simulink model "Test_Aekf"  (R2025b)
settings: Solver=VariableStepAuto  StartTime=0.0  StopTime=StopTime  RelTol=1e-3
undefined symbols (not defined in the file or in its folder): batt
settings Model: Creator=faxio  LastModifiedBy=faxio

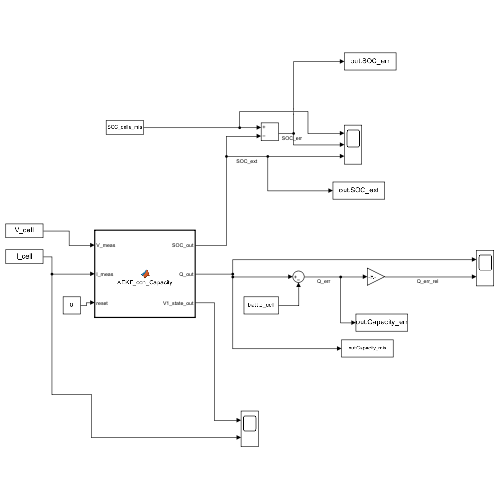
[thumbnail: Simulink's stored preview of the top-level diagram]
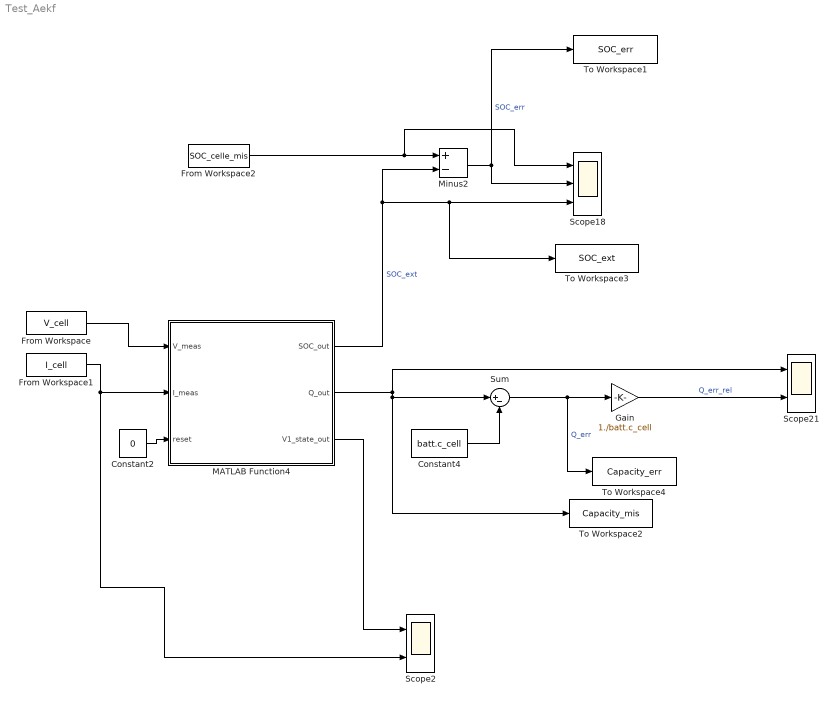
== system Test_Aekf ==
  Constant2 : Constant  Value=0
  Constant4 : Constant  Value=batt.c_cell
  From Workspace : FromWorkspace  VariableName=V_cell
  From Workspace1 : FromWorkspace  VariableName=I_cell
  From Workspace2 : FromWorkspace  VariableName=SOC_celle_mis
  Gain : Gain  Gain=1./batt.c_cell
  MATLAB Function4 : MATLAB Function  TreatAsAtomicUnit=on
  Minus2 : Sum  Inputs=+-
  Scope18 : Scope  NumInputPorts=3
      settings: ActiveDisplayYMinimum=-0.012590051184695097  ActiveDisplayYMaximum=1.1125100056871884  DataLoggingVariableName=ScopeData18
  Scope2 : Scope  NumInputPorts=2
      settings: ActiveDisplayYMinimum=-0.38132934403952395  ActiveDisplayYMaximum=0.3863878602749713
  Scope21 : Scope  NumInputPorts=2
      settings: ActiveDisplayYMinimum=55.008001380546148  ActiveDisplayYMaximum=58.3341308269945  DataLoggingVariableName=ScopeData21
  Sum : Sum  Inputs=|+-
  To Workspace1 : ToWorkspace  VariableName=SOC_err  SaveFormat=Timeseries  SampleTime=-1
  To Workspace2 : ToWorkspace  VariableName=Capacity_mis  SaveFormat=Timeseries  SampleTime=-1
  To Workspace3 : ToWorkspace  VariableName=SOC_ext  SaveFormat=Timeseries  SampleTime=-1
  To Workspace4 : ToWorkspace  VariableName=Capacity_err  SaveFormat=Timeseries  SampleTime=-1
  wires:
  Sum/1 -> To Workspace4/1, Gain/1  "Q_err"
  MATLAB Function4/2(Q_out) -> Scope21/1, To Workspace2/1, Sum/1
  Constant4/1 -> Sum/2
  Constant2/1 -> MATLAB Function4/3(reset)
  MATLAB Function4/1(SOC_out) -> Minus2/2, Scope18/3, To Workspace3/1  "SOC_ext"
  Minus2/1 -> To Workspace1/1, Scope18/2  "SOC_err"
  From Workspace/1 -> MATLAB Function4/1(V_meas)
  From Workspace1/1 -> Scope2/2, MATLAB Function4/2(I_meas)
  From Workspace2/1 -> Scope18/1, Minus2/1
  Gain/1 -> Scope21/2  "Q_err_rel"
  MATLAB Function4/3(V1_state_out) -> Scope2/1

== matlab function Test_Aekf/MATLAB Function4 ==
  settings: updateMethod=DISCRETE  sampleTime=0.5
  data: SOC_out output; Q_out output; V_meas input; I_meas input; reset input; batt_param parameter; V1_state_out output
function [SOC_out, Q_out,V1_state_out]   = AEKF_con_Capacity(V_meas, I_meas, reset,batt_param)  %#codegen

% Ingressi:
%   V_meas - Vettore tensioni misurate [n_cells x 1]
%   I_meas - Vettore correnti misurate [n_cells x 1]  
%   reset  - Segnale di reset (booleano)
%
% Uscita:
%   SOC_out - SOC stimato [n_cells x 1]
%   Q_out   - Capacità stimata [n_cells x 1]


    M=50; %finestra di misura per AEKF
    % Numero di celle 
    n_cells = 4;

    % Parametri batteria
    Ts = 0.5;           % Tempo campionamento [s]
    Q_cell = batt_param.c_cell;        % Capacità nominale [Ah]
    R0_matrix = batt_param.r0;         % Resistenza ohmica [Ohm]
    R1_matrix = batt_param.r1;         % Resistenza RC [Ohm]
    C1_matrix = batt_param.c1;          % Capacità RC [F]
    
    SOC_grid =batt_param.soc(:);
    OCV_tab  =batt_param.ocv(:);
    dOCV_tab =batt_param.docv(:);

    % % Rumore EKF
    % Q_cov = diag([1e-5, 1e-3, 1e-8]);
    % R_var = 0.00001;
    
    persistent SOC_state V1_state Q_state P_state H_k_vector Q_cov R_var initialized 
    persistent I_prev %variabile messa per salvare la corrente precedente e verificare se ci sono picchi di corrente

        if isempty(I_prev)
        I_prev = zeros(n_cells, 1);
        end

    if isempty(initialized) || reset
        SOC_state = 0.5 * ones(n_cells,1);
        V1_state  = zeros(n_cells,1);
        Q_state   = Q_cell(:); % inizializza con capacità nominale
        P_state   = zeros(3,3,n_cells);
    
        %inizializziamo i parametri, uno per ogni cella
        H_k_vector = NaN(n_cells, M); 
        Q_cov = zeros(3, 3, n_cells); 
        R_var = zeros(n_cells, 1);   
    
        for k = 1:n_cells
            P_state(:,:,k) = diag([0.05, 0.01, 1e-3]);

            Q_cov(:,:,k) = diag([1e-5, 1e-3, 1e-10]); % rumore piccolo inizialmente su Q (variazione lenta)
            R_var(k) = 0.00001;
        end
        initialized = true;
    end

    %% PRE-ALLOCAZIONE

    SOC_out = zeros(n_cells,1);
    Q_out   = zeros(n_cells,1);

    V1_state_out= zeros(n_cells,1);


    %% EKF PER OGNI CELLA

    for k = 1:n_cells

        % Stato corrente
        x = [SOC_state(k); V1_state(k); Q_state(k)];
        P = P_state(:,:,k);

        Q_cov_k = Q_cov(:,:,k);  
        R_var_k = R_var(k);

        I_k = I_meas(k);
        V_k = V_meas(k);

        %% PREDIZIONE 
        % Coulomb counting
        Q_k = max(1e-6, x(3)); % fa evitare divisione per zero
        SOC_pred = x(1) - (Ts * I_k) / (Q_k * 3600);
        SOC_pred = max(0.1, min(1, SOC_pred)); %limito il soc tra 0.1 e 1
    
        % ESTRAGGO LA RIGA k DALLA MATRICE E FACCIO L'INTERPOLAZIONE
        R0_row = R0_matrix(k, :);  % Riga k, vettore [1 x 21]
        R1_row = R1_matrix(k, :);  % Riga k, vettore [1 x 21]
        C1_row = C1_matrix(k, :);  % Riga k, vettore [1 x 21]
        
        % Converte a colonna per interp1
        R0_col = R0_row(:);  % [21 x 1]
        R1_col = R1_row(:);  % [21 x 1]
        C1_col = C1_row(:);  % [21 x 1]

        % Interpolazione
        R0 = interp1(SOC_grid, R0_col, SOC_pred, 'linear', 'extrap');
        R1 = interp1(SOC_grid, R1_col, SOC_pred, 'linear', 'extrap');
        C1 = interp1(SOC_grid, C1_col, SOC_pred, 'linear', 'extrap');
    
        R0=R0/Q_k*Q_cell(k);
        R1=R1/Q_k*Q_cell(k);
        C1=C1*Q_k/Q_cell(k);

        tau1  = R1 * C1;
        alpha = exp(-Ts / tau1);

        % Dinamica RC
        V1_pred = alpha * x(2) + R1 * (1 - alpha) * I_k;

        % Q pred
        Q_pred = x(3);

        x_pred = [SOC_pred; V1_pred; Q_pred];

        % Jacobiano stato
        dSOCdQ = (Ts * I_k) / (Q_k^2 * 3600);
        A =[1, 0, dSOCdQ;
            0, alpha, 0;
            0, 0, 1];
        
        %% ///////////////////////////////////
        % inserisco una condizione che verifica che la derivata della
        % corrente non sia molto alta, nel caso in cui lo fosse Q_cov va
        % aumentato. Ho aggiunto come persistent Iprev
        

        % Rileviamo la variazione di corrente
        dI = abs(I_k - I_prev(k));

        if dI > 0.3 * Q_cell(k)  % Impulso rilevato
            Q_cov_k_temp = Q_cov_k;
            Q_cov_k_temp(1,1) = Q_cov_k(1,1) * 100;
            Q_cov_k_temp(2,2) = Q_cov_k(2,2) * 50;  
            % Q(3,3) rimane uguale (variazione di capacità lenta)
        else
            Q_cov_k_temp = Q_cov_k;  %// Usa valore normale
        end

        P_pred = A * P * A' + Q_cov_k_temp;

        I_prev(k) = I_k;

        %////////////////////////////////////////
        %% AGGIORNAMENTO
        OCV  = interp1(SOC_grid, OCV_tab, SOC_pred,"linear","extrap");
        dOCV = interp1(SOC_grid, dOCV_tab, SOC_pred,"linear","extrap");
        
        V_pred = OCV - x_pred(2) - R0 * I_k;
        y_tilde = V_k - V_pred;
    
        %liomitiamo per swicurezza anche y_tilde soprattutto ad alte correnti
        C_rate = abs(I_k) / Q_cell(k);
        if C_rate > 1.5
            y_tilde = max(-0.1, min(0.1, y_tilde));
        else
            y_tilde = max(-0.8, min(0.8, y_tilde));
        end

        C_mat = [dOCV, -1, 0];

        S = C_mat * P_pred * C_mat' + R_var_k;
        K = (P_pred * C_mat') / S;
        
        % Possiamo pensare di inserire una protezione sulla stima della
        % capacità per far in modo che venga più precisa mettendo dei
        % limitti su quando stimarla.

        % Condizioni per NON aggiornare Q:
        disable_Q_update = false;

        % 1. Corrente troppo bassa (< 0.1C)
        if abs(I_k) < 0.1 * Q_cell(k)
            disable_Q_update = true;
        end

        % 2. Picchi di corrente
        if dI > 0.3 * Q_cell(k)
            disable_Q_update = true;
        end

        % 3. SOC estremi (modello impreciso)
        if SOC_pred < 0.15 || SOC_pred > 0.85
            disable_Q_update = true;
        end

        % 4. Innovazione troppo grande (modello sbagliato)
        if abs(y_tilde) > 0.1
            disable_Q_update = true;
        end

        % Azzera K(3) se le condizioni non sono buone
        if disable_Q_update
            K(3) = 0; 
        end
        %%

        % Aggiornamento stato
        x_upd = x_pred + K * y_tilde;
        x_upd(1) = max(0.05, min(1, x_upd(1)));
        x_upd(3) = max(1e-6, x_upd(3)); % capacità sempre positiva

        % Aggiornamento covarianza
        I3 = eye(3);
        P_upd = (I3 - K * C_mat) * P_pred;

        % Forziamo la simmetria
        P_upd = (P_upd + P_upd') / 2;

        H_k_vector(k,:)=circshift(H_k_vector(k,:),1);
        H_k_vector(k,1)=y_tilde*y_tilde';
        if ~isnan(H_k_vector(k,M))
            H_k=sum(H_k_vector(k,:))/M;
        
            %visto che a volte diverge, proviamo ad impostare dei limiti su Q ed R_var
            Q_cov_k_new=K * H_k * K';
        
            %facciamo in modo che sia una matrice simmetrica
            Q_cov_k_new = (Q_cov_k_new + Q_cov_k_new') / 2;

            Q_limits_min = [1e-12; 1e-10; 1e-12]; 
            Q_limits_max = [1e-2; 1e-2; 1e-2]; 
            for i = 1:3
                Q_cov_k_new(i,i) = max(Q_limits_min(i), min(Q_limits_max(i), Q_cov_k_new(i,i)));
            end
        
            Q_cov_k=0.8 * Q_cov_k + 0.2 * Q_cov_k_new; %aggiornamento lento
        
            % impostiamo dei limiti anche su R_var
            R_var_k_new=H_k-C_mat*P_upd*C_mat';

            if R_var_k_new > 0
                R_var_k_new = max(1e-6, min(0.1, R_var_k_new)); % Clamp
                % Aggiornamento lento per stabilità
                R_var_k = 0.8 * R_var_k + 0.2 * R_var_k_new;
            else
                % Se negativo, aumenta lentamente verso valore sicuro
                R_var_k = 0.95 * R_var_k + 0.05 * 1e-6;
            end
       
        end

        Qmin = 0.4 * Q_cell(k);
        Qmax = 1.1 * Q_cell(k);
        x_upd(3) = min(Qmax, max(Qmin, x_upd(3)));

        %% SALVATAGGIO 
        SOC_state(k) = x_upd(1);
        V1_state(k)  = x_upd(2);
        Q_state(k)   = x_upd(3);
        P_state(:,:,k) = P_upd;
        Q_cov(:,:,k) = Q_cov_k;
        R_var(k)=R_var_k;
    
        %% OUTPUT
        SOC_out(k) = x_upd(1);
        Q_out(k)   = x_upd(3);
        V1_state_out(k)=x_upd(2);

    end
end
